simulink model "expe2_model_v2"  (R2019b)
settings: Solver=VariableStepAuto  StartTime=0.0  StopTime=time  RelTol=1e-3
values from neighbouring files (symbols this model uses):
  system1 = ModelPID(a1, a2, b0, b1, damp_coeff1, wn1, lambda)    [expe2_params.m]
settings Model: Creator=adityaaaap  LastModifiedBy=adityaaaap

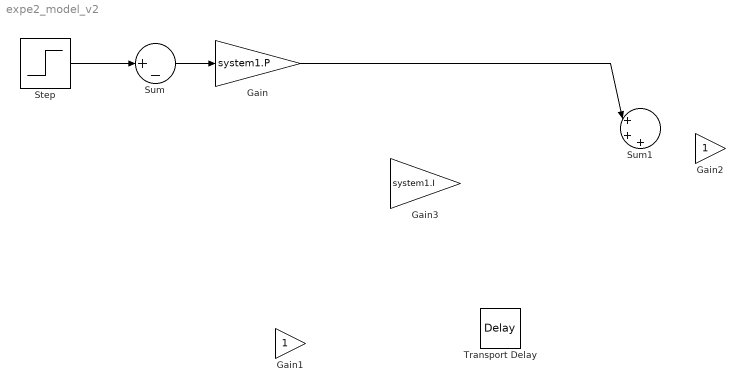
== system expe2_model_v2 ==
  Gain : Gain  Gain=system1.P
  Gain1 : Gain
  Gain2 : Gain
  Gain3 : Gain  Gain=system1.I
  Step : Step  Time=0  After=3  SampleTime=0.1
  Sum : Sum  Inputs=|+-
  Sum1 : Sum  Inputs=|+++
  Transport Delay : TransportDelay
  wires:
  Step/1 -> Sum/1
  Sum/1 -> Gain/1
  Gain/1 -> Sum1/1
